simulink model "linearized_system_question_3"  (R2023b)
settings: Solver=VariableStepAuto  StartTime=0.0  StopTime=100.0  RelTol=1e-3
settings Model: Creator=orife  LastModifiedBy=orife

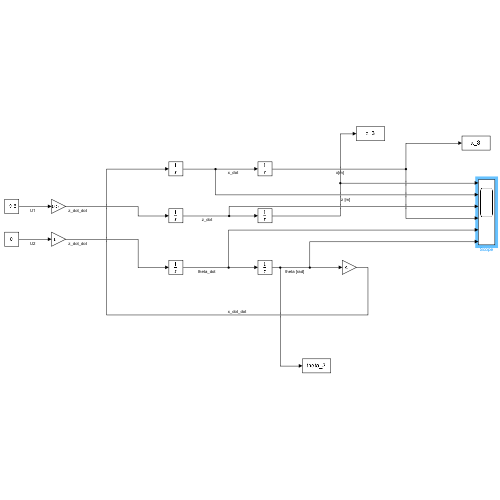
[thumbnail: Simulink's stored preview of the top-level diagram]
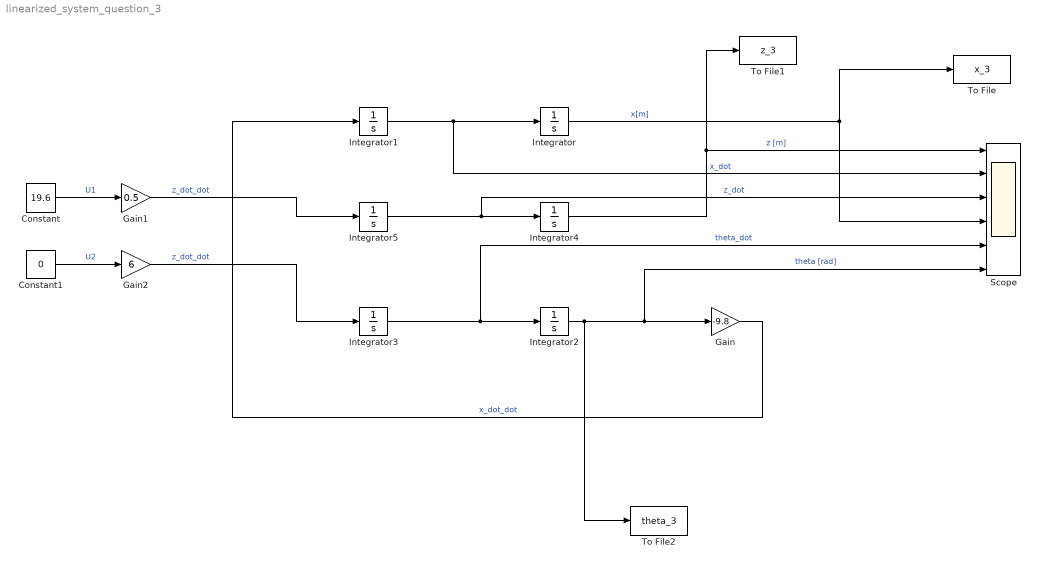
== system linearized_system_question_3 ==
  Constant : Constant  Value=19.6
  Constant1 : Constant  Value=0
  Gain : Gain  Gain=-9.8
  Gain1 : Gain  Gain=0.5
  Gain2 : Gain  Gain=6
  Integrator{,1,3..5} (5 alike) : Integrator
  Integrator2 : Integrator  InitialCondition=(4/180)*pi
  Scope : Scope  NumInputPorts=6
  To File : ToFile  Filename=x_3  SaveFormat=Timeseries
  To File1 : ToFile  Filename=z_3  SaveFormat=Timeseries
  To File2 : ToFile  Filename=theta_3  SaveFormat=Timeseries
  wires:
  Integrator1/1 -> Scope/2, Integrator/1  "x_dot"
  Integrator3/1 -> Scope/5, Integrator2/1  "theta_dot"
  Integrator5/1 -> Scope/3, Integrator4/1  "z_dot"
  Integrator2/1 -> To File2/1, Scope/6, Gain/1  "theta [rad]"
  Gain/1 -> Integrator1/1  "x_dot_dot"
  Gain1/1 -> Integrator5/1  "z_dot_dot"
  Constant/1 -> Gain1/1  "U1"
  Constant1/1 -> Gain2/1  "U2"
  Gain2/1 -> Integrator3/1  "z_dot_dot"
  Integrator4/1 -> To File1/1, Scope/1  "z [m]"
  Integrator/1 -> To File/1, Scope/4  "x[m]"
